simulink model "fig_8_14"  (R2022a)
settings: Solver=ode8  StartTime=0.0  StopTime=30  FixedStep=0.001  RelTol=1e-3
settings Model: Creator=wdrac  LastModifiedBy=wdrac

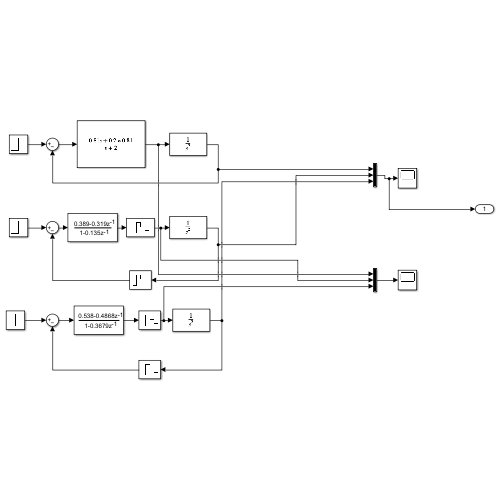
[thumbnail: Simulink's stored preview of the top-level diagram]
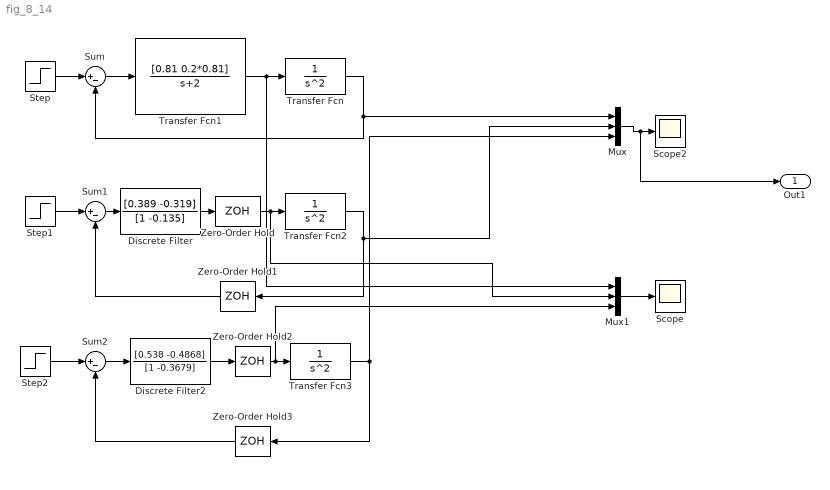
== system fig_8_14 ==
  Discrete Filter : DiscreteFilter  Numerator=[0.389 -0.319]  Denominator=[1 -0.135]  SampleTime=1
  Discrete Filter2 : DiscreteFilter  Numerator=[0.538 -0.4868]  Denominator=[1 -0.3679]  SampleTime=0.5
  Mux : Mux  Inputs=3
  Mux1 : Mux  Inputs=3
  Scope : Scope
  Scope2 : Scope
  Step : Step  Before=1  SampleTime=0
  Step1 : Step  Before=1  SampleTime=0
  Step2 : Step  Before=1  SampleTime=0.5
  Sum : Sum  Inputs=|+-
  Sum1 : Sum  Inputs=|+-
  Sum2 : Sum  Inputs=|+-
  Transfer Fcn : TransferFcn  Denominator=[1 0 0]
  Transfer Fcn1 : TransferFcn  Numerator=[0.81 0.2*0.81]  Denominator=[1 2]
  Transfer Fcn2 : TransferFcn  Denominator=[1 0 0]
  Transfer Fcn3 : TransferFcn  Denominator=[1 0 0]
  Zero-Order Hold : ZeroOrderHold
  Zero-Order Hold1 : ZeroOrderHold
  Zero-Order Hold2 : ZeroOrderHold  SampleTime=0.5
  Zero-Order Hold3 : ZeroOrderHold  SampleTime=0.5
  Out1 : Outport
  wires:
  Transfer Fcn1/1 -> Mux1/1, Transfer Fcn/1
  Transfer Fcn/1 -> Mux/1, Sum/2
  Step/1 -> Sum/1
  Sum/1 -> Transfer Fcn1/1
  Transfer Fcn2/1 -> Mux/2, Zero-Order Hold1/1
  Step1/1 -> Sum1/1
  Zero-Order Hold/1 -> Mux1/2, Transfer Fcn2/1
  Zero-Order Hold1/1 -> Sum1/2
  Sum1/1 -> Discrete Filter/1
  Discrete Filter/1 -> Zero-Order Hold/1
  Mux/1 -> Out1/1, Scope2/1
  Mux1/1 -> Scope/1
  Sum2/1 -> Discrete Filter2/1
  Step2/1 -> Sum2/1
  Transfer Fcn3/1 -> Zero-Order Hold3/1, Mux/3
  Zero-Order Hold2/1 -> Mux1/3, Transfer Fcn3/1
  Zero-Order Hold3/1 -> Sum2/2
  Discrete Filter2/1 -> Zero-Order Hold2/1
